simulink model "top_model"  (R2019b)
settings: Solver=VariableStepAuto  StartTime=0.0  StopTime=10  RelTol=1e-3
model workspace (MAT data in the model file):
  CDen = [1 0]
  CNum = [0.566666666667 1.19]
  J = 0.02
  Kb = 0.1
  Kf = 0.2
  Ki = 4.051
  Km = 0.1
  Kp = 1.653
  L = 0.5
  R = 2
libraries: simulink x1
settings Model: OrderedModelArguments=off  Creator=cleme  LastModifiedBy=cleme
settings DataIOCC: ReturnWorkspaceOutputs=off
settings DebuggingCC: ArithmeticOperatorsInVariantConditions=warning
settings SFSimCC: CustomCodeUndefinedFunction=UseInterfaceOnly

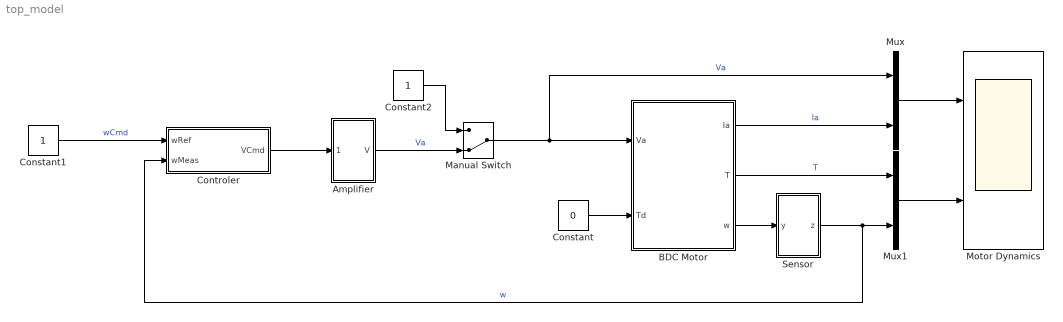
== system top_model ==
  Amplifier : Subsystem
  BDC Motor : Subsystem
  Constant : Constant  Value=0
  Constant1 : Constant
  Constant2 : Constant
  Controler : Subsystem
  Manual Switch : ManualSwitch  CurrentSetting=0
  Motor Dynamics : Scope  NumInputPorts=2
  Mux : Mux  Inputs=2
  Mux1 : Mux  Inputs=2
  Sensor : Subsystem
  wires:
  Constant/1 -> BDC Motor/2(Td)
  Sensor/1(z) -> Controler/2(wMeas), Mux1/2  "w"
  BDC Motor/3(w) -> Sensor/1(y)
  Controler/1(VCmd) -> Amplifier/1(PWM)
  Manual Switch/1 -> Mux/1, BDC Motor/1(Va)  "Va"
  Constant1/1 -> Controler/1(wRef)  "wCmd"
  Mux/1 -> Motor Dynamics/1
  Mux1/1 -> Motor Dynamics/2
  BDC Motor/1(Ia) -> Mux/2  "Ia"
  BDC Motor/2(T) -> Mux1/1  "T"
  Amplifier/1(V) -> Manual Switch/2  "Va"
  Constant2/1 -> Manual Switch/1

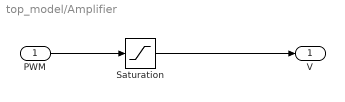
== system top_model/Amplifier ==
  PWM : Inport  Unit=V
  Saturation : Saturate  UpperLimit=10  LowerLimit=-10
  V : Outport  Unit=V  VectorParamsAs1DForOutWhenUnconnected=off
  wires:
  PWM/1 -> Saturation/1
  Saturation/1 -> V/1

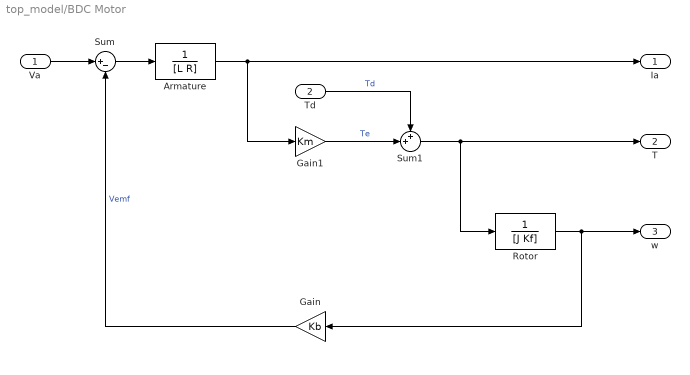
== system top_model/BDC Motor ==
  Va : Inport  Unit=V
  Td : Inport  Port=2  Unit=N*m
  Armature : TransferFcn  Numerator=1  Denominator=[L R]
  Gain : Gain  Gain=Kb
  Gain1 : Gain  Gain=Km
  Rotor : TransferFcn  Denominator=[J Kf]
  Sum : Sum  Inputs=|+-
  Sum1 : Sum  Inputs=++|
  Ia : Outport
  T : Outport  Port=2
  w : Outport  Port=3  Unit=rad/s  VectorParamsAs1DForOutWhenUnconnected=off
  wires:
  Sum1/1 -> Rotor/1, T/1
  Sum/1 -> Armature/1
  Va/1 -> Sum/1
  Rotor/1 -> w/1, Gain/1
  Td/1 -> Sum1/1  "Td"
  Gain/1 -> Sum/2  "Vemf"
  Armature/1 -> Ia/1, Gain1/1
  Gain1/1 -> Sum1/2  "Te"

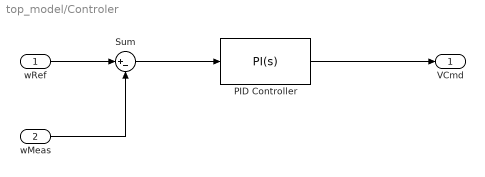
== system top_model/Controler ==
  wRef : Inport  Unit=rad/s
  wMeas : Inport  Port=2  Unit=rad/s
  PID Controller : simulink/Continuous/PID Controller  Controller=PI  Form=Parallel  TimeDomain=Continuous-time  SampleTime=-1  IntegratorMethod=Forward Euler  FilterMethod=Forward Euler  ControllerParametersSource=internal  P=Kp  I=Ki  D=0  UseFilter=on  N=100  TunerSelectOption=Transfer Function Based (PID Tuner App)  InitialConditionSource=internal  InitialConditionForIntegrator=0  InitialConditionForFilter=0  DifferentiatorICPrevScaledInput=0  ExternalReset=none  TrackingMode=off  Kt=1  LimitOutput=on  UpperSaturationLimit=10  LowerSaturationLimit=-10  LinearizeAsGain=on  AntiWindupMode=back-calculation  Kb=Ki  POutMin=[]  POutMax=[]  IOutMin=[]  IOutMax=[]  DOutMin=[]  DOutMax=[]  NOutMin=[]  NOutMax=[]  SumOutMin=[]  SumOutMax=[]  SaturationOutMin=[]  SaturationOutMax=[]  PParamMin=[]  PParamMax=[]  IParamMin=[]  IParamMax=[]  DParamMin=[]  DParamMax=[]  NParamMin=[]  NParamMax=[]  KbParamMin=[]  KbParamMax=[]  KtParamMin=[]  KtParamMax=[]  KbOutMin=[]  KbOutMax=[]  KtOutMin=[]  KtOutMax=[]  IntegratorOutMin=[]  IntegratorOutMax=[]  FilterOutMin=[]  FilterOutMax=[]  SumI1OutMin=[]  SumI1OutMax=[]  SumI2OutMin=[]  SumI2OutMax=[]  SumI3OutMin=[]  SumI3OutMax=[]  SumI4OutMin=[]  SumI4OutMax=[]  SumDOutMin=[]  SumDOutMax=[]  DifferentiatorOutMin=[]  DifferentiatorOutMax=[]  FilterDiffOutCoefMin=[]  FilterDiffOutCoefMax=[]  ReciprocalOutMin=[]  ReciprocalOutMax=[]  SumDenOutMin=[]  SumDenOutMax=[]  SumNumOutMin=[]  SumNumOutMax=[]  DivideOutMin=[]  DivideOutMax=[]  IntegratorContinuousStateAttributes=''  IntegratorStateMustResolveToSignalObject=off  IntegratorRTWStateStorageClass=Auto  FilterContinuousStateAttributes=''  FilterStateMustResolveToSignalObject=off  FilterRTWStateStorageClass=Auto  ParallelPVariant=InternalParameters  IdealPVariant=Disabled  IVariant=InternalParameters  DVariant=Disabled  IntegratorVariant=Continuous  SatVariant=Enabled  AWVariant=BackCalculation  PCopyVariant=Disabled  TRVariant=Disabled  FdbkBlocksVariant=Forward  IdealPFdbkVariant=Disabled  SatFdbkVariant=Disabled  DerivativeFilterVariant=Disabled  NVariant=Disabled  NCopyVariant=Disabled_SignalSpec  FilterICVariant=Disabled  IntegratorICVariant=InternalICs  ExternalResetVariant=Disabled  TRSumVariant=Passthrough  SumFdbkVariant=Disabled  SumVariant=Sum_PI
  Sum : Sum  Inputs=|+-
  VCmd : Outport  Unit=V  VectorParamsAs1DForOutWhenUnconnected=off
  wires:
  wRef/1 -> Sum/1
  wMeas/1 -> Sum/2
  Sum/1 -> PID Controller/1
  PID Controller/1 -> VCmd/1

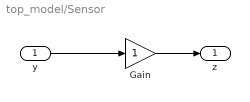
== system top_model/Sensor ==
  y : Inport  Unit=rad/s
  Gain : Gain
  z : Outport  Unit=rad/s  VectorParamsAs1DForOutWhenUnconnected=off
  wires:
  y/1 -> Gain/1
  Gain/1 -> z/1
